simulink library "Lib_Turbo_Splitter_TMATS"  (R2015a)
settings: Solver=ode45  StartTime=0.0  StopTime=10.0  RelTol=1e-3
Description:
  | Thomas Modules
settings Model: Creator=jwchapm2  LastModifiedBy=jwchapm2
settings OptimizationCC: ExpressionDepthLimit=2147483647
settings DebuggingCC: UnderspecifiedInitializationDetection=Classic  MergeDetectMultiDrivingBlocksExec=none  SolverPrmCheckMsg=warning  StateNameClashWarn=warning

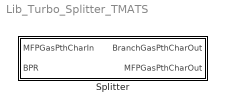
== system Lib_Turbo_Splitter_TMATS ==
  Splitter : Subsystem  mask(T-MATS: Splitter Library Block){}
      mask help: This block simulates the performance of a splitter/branch using basic flow relationships.
      mask Help: web(which('Turbo_TMATS_Splt.html'),'-helpbrowser')

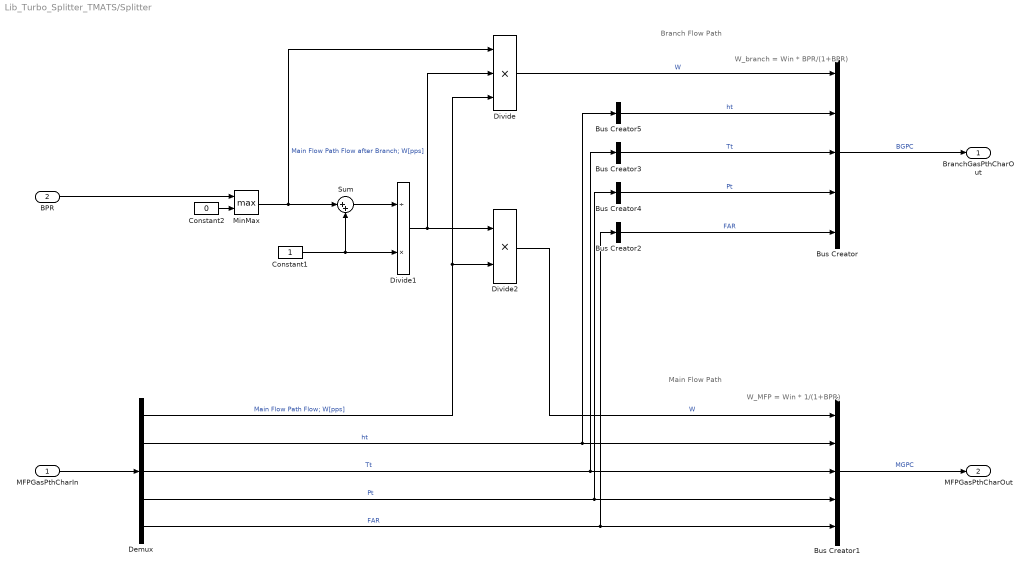
== system Lib_Turbo_Splitter_TMATS/Splitter ==
  note: Main Flow Path
  note: W_branch = Win * BPR/(1+BPR)
  note: W_MFP = Win * 1/(1+BPR)
  note: Branch Flow Path
  MFPGasPthCharIn : Inport
  BPR : Inport  Port=2
  Bus Creator : BusCreator  Inputs=5
  Bus Creator1 : BusCreator  Inputs=5
  Bus Creator{2..5} (4 alike) : BusCreator  Inputs=1
  Constant1 : Constant
  Constant2 : Constant  Value=0
  Demux : Demux  Outputs=5
  Divide : Product  Inputs=***
  Divide1 : Product  Inputs=/*
  Divide2 : Product  Inputs=**
  MinMax : MinMax  Function=max  Inputs=2
  Sum : Sum  Inputs=|++
  BranchGasPthCharOut : Outport
  MFPGasPthCharOut : Outport  Port=2
  wires:
  Bus Creator/1 -> BranchGasPthCharOut/1  "BGPC"
  Demux/4 -> Bus Creator4/1, Bus Creator1/4  "Pt"
  Demux/3 -> Bus Creator3/1, Bus Creator1/3  "Tt"
  Demux/5 -> Bus Creator2/1, Bus Creator1/5  "FAR"
  MFPGasPthCharIn/1 -> Demux/1
  Bus Creator1/1 -> MFPGasPthCharOut/1  "MGPC"
  Constant1/1 -> Sum/2, Divide1/2
  Divide2/1 -> Bus Creator1/1  "W"
  Divide/1 -> Bus Creator/1  "W"
  Bus Creator2/1 -> Bus Creator/5  "FAR"
  Bus Creator3/1 -> Bus Creator/3  "Tt"
  Bus Creator4/1 -> Bus Creator/4  "Pt"
  Sum/1 -> Divide1/1
  Demux/1 -> Divide/3, Divide2/2  "Main Flow Path Flow; W[pps]"
  Divide1/1 -> Divide/2, Divide2/1  "Main Flow Path Flow after Branch; W[pps]"
  Demux/2 -> Bus Creator5/1, Bus Creator1/2  "ht"
  Bus Creator5/1 -> Bus Creator/2  "ht"
  MinMax/1 -> Divide/1, Sum/1
  Constant2/1 -> MinMax/2
  BPR/1 -> MinMax/1
